simulink library "lib_fuel_converter3"  (Simulink 4.1.1)
values from neighbouring files (symbols this model uses):
  logFlag = 1    [advSACompMaskInit.m]    (also in advSACompMaskInitR13.m)
undefined symbols (not defined in the file or in its folder): air_cp, amb_tmp, cyc_mph, ex_gas_cp, fc_acc_mass, fc_base_mass, fc_c2i_th_cond, fc_c_init_tmp, fc_cl2h_eff, fc_CO2_to_FUELgps, fc_cold, fc_cold_tmp, fc_cp, fc_ct_trq, fc_emisv, fc_ext_sarea, fc_fuel_den, fc_fuel_lhv, fc_h2x_th_cond, fc_h_air_flow, fc_h_cp, fc_h_init_tmp, fc_hood_emisv, fc_hood_sarea, fc_i2x_th_cond, fc_i_init_tmp, fc_inertia, fc_map_spd, fc_map_trq, fc_max_trq, fc_nn_model_name, fc_pwr_scale, fc_spd_scale, fc_trq_scale, fc_tstat, fc_x_init_tmp, fd_ratio, gb_num_init, gb_ratio, generalName, pow, vc_idle_bool, vc_idle_spd, vc_key_on, veh_glider_mass, wh_radius
libraries: lib_fuel_converter3 x4, lib_etc x4, lib_fuel_converter x2, lib_fuel_converter2 x1
(part 4 of 9)

== system lib_fuel_converter3/configurable subsystems/fuel use and EO emis/fc temp/old fc coolant  temp. (C) ==
  fc on? : Inport  Port=1  LatchInput=off
  veh spd : Inport  Port=2  LatchInput=off
  Block NOTES : Subsystem
      settings: RTWFcnNameOpts=Auto  RTWFileNameOpts=Auto
      mask Display: disp('Block\nNOTES')
  Mux : Mux  Inputs=4
      settings: DisplayOption=none
  TEC : Integrator  ExternalReset=none  InitialConditionSource=internal  InitialCondition=fc_i_init_tmp  LimitOutput=off  UpperSaturationLimit=inf  LowerSaturationLimit=-inf  ShowSaturationPort=off  ShowStatePort=off  AbsoluteTolerance=auto
  compute engine dT/dt : Fcn  Expr=1.1*u[1]*(-u[2]/218)*(95-u[4])+(1-u[1])*u[3]*(u[4]-amb_tmp)
  gamma (takes v as input) : Fcn  Expr=(-8.22e-5*u+8.09e-6*4-1.45e-4)*.45
  log(1-40/75) : Constant  Value=-0.7621
  fc coolant  temp (C) : Outport  Port=1  InitialOutput=0
  wires:
  compute engine dT/dt/1 -> TEC/1
  gamma (takes v as input)/1 -> Mux/3
  log(1-40/75)/1 -> Mux/2
  Mux/1 -> compute engine dT/dt/1
  fc on?/1 -> Mux/1
  veh spd/1 -> gamma (takes v as input)/1
  TEC/1 -> fc coolant  temp (C)/1, Mux/4

== system lib_fuel_converter3/configurable subsystems/fuel use and EO emis/fc temp correct/fc temp correct Constant Correction Factors (Equation Based) ==
  Coolant T (C) : Inport  Port=1  LatchInput=off
  HOT fuel use (g/s) : Inport  Port=2  LatchInput=off
  HOT emis (g/s) : Inport  Port=3  LatchInput=off
  Enable : EnablePort  StatesWhenEnabling=reset
  Block NOTES : Subsystem
      settings: RTWFcnNameOpts=Auto  RTWFileNameOpts=Auto
      mask Display: disp('Block\nNOTES')
  CO cold/hot : Fcn  Expr=2.13*pow(u,4.26)+1
  HC cold/hot : Fcn  Expr=8.05*pow(u,9.46)+1
  Mux : Mux  Inputs=4
      settings: DisplayOption=none
  NOx cold/hot : Fcn  Expr=0.51*pow(u,1.37)+1
  PM cold/hot : Fcn  Expr=5.14*pow(u,17.04)+1
  Product : Product  Inputs=2  Multiplication=Element-wise(.*)  SaturateOnIntegerOverflow=on
  Product1 : Product  Inputs=2  Multiplication=Element-wise(.*)  SaturateOnIntegerOverflow=on
  Saturation : Saturate  UpperLimit=1  LowerLimit=0  LinearizeAsGain=on
  fuel cold/hot : Fcn  Expr=0.1*pow(u,0.65)+1
  lambda : Fcn  Expr=(fc_tstat-u)/(fc_tstat-20)
  fuel use (g/s) : Outport  Port=1  OutputWhenDisabled=reset  InitialOutput=0
  EO emis (g/s) : Outport  Port=2  OutputWhenDisabled=reset  InitialOutput=0
  wires:
  PM cold/hot/1 -> Mux/4
  NOx cold/hot/1 -> Mux/3
  HC cold/hot/1 -> Mux/1
  Saturation/1 -> CO cold/hot/1, HC cold/hot/1, fuel cold/hot/1, NOx cold/hot/1, PM cold/hot/1
  lambda/1 -> Saturation/1
  Mux/1 -> Product/1
  fuel cold/hot/1 -> Product1/2
  Product/1 -> EO emis (g/s)/1
  CO cold/hot/1 -> Mux/2
  Product1/1 -> fuel use (g/s)/1
  HOT fuel use (g/s)/1 -> Product1/1
  Coolant T (C)/1 -> lambda/1
  HOT emis (g/s)/1 -> Product/2

== system lib_fuel_converter3/configurable subsystems/fuel use and EO emis/fc temp correct/fc temp correct Variable Correction Factors (Map Based) ==
  Coolant T (C) : Inport  Port=1  LatchInput=off
  HOT fuel use (g/s) : Inport  Port=2  LatchInput=off
  HOT emis (g/s) : Inport  Port=3  LatchInput=off
  T (Nm) : Inport  Port=4  LatchInput=off
  w (rad/s) : Inport  Port=5  LatchInput=off
  Enable : EnablePort  StatesWhenEnabling=reset
  (Thot-Temp) -------------------- (Thot-Tcold) : Fcn  Expr=(fc_tstat-u)/(fc_tstat-fc_cold_tmp)
  CO factor cold-to-hot : Subsystem  mask(2-D Table Lookup){@1=fc_map_spd*fc_spd_scale, @2=fc_map_trq*fc_trq_scale, @3=fc_co_map_c2h}
      mask prompts: @1 "X Index"; @2 "Y Index"; @3 "Table"
      mask help:
      | Two Dimensional Table Lookup
      | The first input corresponds to X Index and the second input corresponds to the Y Index
      mask init:
      | xindex=@1; yindex=@2; table=@3; sftab2chk(xindex,yindex,table);
      settings: RTWFcnNameOpts=Auto  RTWFileNameOpts=Auto
      mask Help: This block returns a linearly interpolated intersection from the table using the X index (which corresponds to the rows of the table) and the Y index (which corresponds to the columns of the table).  Extrapolation is used.
      mask Display: plot(-10,-10,110,110,[90,50,10],[90,40,30],[90,50,10],[50,26,20],[90,50,10],[22,13,10])
  HC factor cold-to-hot : Subsystem  mask(2-D Table Lookup){@1=fc_map_spd*fc_spd_scale, @2=fc_map_trq*fc_trq_scale, @3=fc_hc_map_c2h}
      mask prompts: @1 "X Index"; @2 "Y Index"; @3 "Table"
      mask help:
      | Two Dimensional Table Lookup
      | The first input corresponds to X Index and the second input corresponds to the Y Index
      mask init:
      | xindex=@1; yindex=@2; table=@3; sftab2chk(xindex,yindex,table);
      settings: RTWFcnNameOpts=Auto  RTWFileNameOpts=Auto
      mask Help: This block returns a linearly interpolated intersection from the table using the X index (which corresponds to the rows of the table) and the Y index (which corresponds to the columns of the table).  Extrapolation is used.
      mask Display: plot(-10,-10,110,110,[90,50,10],[90,40,30],[90,50,10],[50,26,20],[90,50,10],[22,13,10])
  Mux{1..5} (5 alike) : Mux  Inputs=2
      settings: DisplayOption=none
  Mux6 : Mux  Inputs=4
      settings: DisplayOption=none
  NOx factor cold-to-hot : Subsystem  mask(2-D Table Lookup){@1=fc_map_spd*fc_spd_scale, @2=fc_map_trq*fc_trq_scale, @3=fc_nox_map_c2h}
      mask prompts: @1 "X Index"; @2 "Y Index"; @3 "Table"
      mask help:
      | Two Dimensional Table Lookup
      | The first input corresponds to X Index and the second input corresponds to the Y Index
      mask init:
      | xindex=@1; yindex=@2; table=@3; sftab2chk(xindex,yindex,table);
      settings: RTWFcnNameOpts=Auto  RTWFileNameOpts=Auto
      mask Help: This block returns a linearly interpolated intersection from the table using the X index (which corresponds to the rows of the table) and the Y index (which corresponds to the columns of the table).  Extrapolation is used.
      mask Display: plot(-10,-10,110,110,[90,50,10],[90,40,30],[90,50,10],[50,26,20],[90,50,10],[22,13,10])
  PM factor cold-to-hot : Subsystem  mask(2-D Table Lookup){@1=fc_map_spd*fc_spd_scale, @2=fc_map_trq*fc_trq_scale, @3=fc_pm_map_c2h}
      mask prompts: @1 "X Index"; @2 "Y Index"; @3 "Table"
      mask help:
      | Two Dimensional Table Lookup
      | The first input corresponds to X Index and the second input corresponds to the Y Index
      mask init:
      | xindex=@1; yindex=@2; table=@3; sftab2chk(xindex,yindex,table);
      settings: RTWFcnNameOpts=Auto  RTWFileNameOpts=Auto
      mask Help: This block returns a linearly interpolated intersection from the table using the X index (which corresponds to the rows of the table) and the Y index (which corresponds to the columns of the table).  Extrapolation is used.
      mask Display: plot(-10,-10,110,110,[90,50,10],[90,40,30],[90,50,10],[50,26,20],[90,50,10],[22,13,10])
  Product : Product  Inputs=2  Multiplication=Element-wise(.*)  SaturateOnIntegerOverflow=on
  Product1 : Product  Inputs=2  Multiplication=Element-wise(.*)  SaturateOnIntegerOverflow=on
  Saturation1 : Saturate  UpperLimit=max(fc_map_trq*fc_trq_scale)  LowerLimit=min(fc_map_trq*fc_trq_scale)  LinearizeAsGain=on
  Saturation2 : Saturate  UpperLimit=max(fc_map_spd*fc_spd_scale)  LowerLimit=min(fc_map_spd*fc_spd_scale)  LinearizeAsGain=on
  cold/hot =1+(factor-1) *Temp_ratio{,1..4} (5 alike) : Fcn  Expr=1+(u[2]-1)*u[1]
  fuel factor cold-to-hot : Subsystem  mask(2-D Table Lookup){@1=fc_map_spd*fc_spd_scale, @2=fc_map_trq*fc_trq_scale, @3=fc_fuel_map_c2h}
      mask prompts: @1 "X Index"; @2 "Y Index"; @3 "Table"
      mask help:
      | Two Dimensional Table Lookup
      | The first input corresponds to X Index and the second input corresponds to the Y Index
      mask init:
      | xindex=@1; yindex=@2; table=@3; sftab2chk(xindex,yindex,table);
      settings: RTWFcnNameOpts=Auto  RTWFileNameOpts=Auto
      mask Help: This block returns a linearly interpolated intersection from the table using the X index (which corresponds to the rows of the table) and the Y index (which corresponds to the columns of the table).  Extrapolation is used.
      mask Display: plot(-10,-10,110,110,[90,50,10],[90,40,30],[90,50,10],[50,26,20],[90,50,10],[22,13,10])
  limit to data limits : Saturate  UpperLimit=1  LowerLimit=0  LinearizeAsGain=on
  fuel use (g/s) : Outport  Port=1  OutputWhenDisabled=reset  InitialOutput=0
  EO emis (g/s) : Outport  Port=2  OutputWhenDisabled=reset  InitialOutput=0
  wires:
  cold/hot =1+(factor-1) *Temp_ratio4/1 -> Mux6/4
  cold/hot =1+(factor-1) *Temp_ratio3/1 -> Mux6/3
  cold/hot =1+(factor-1) *Temp_ratio2/1 -> Mux6/2
  cold/hot =1+(factor-1) *Temp_ratio1/1 -> Mux6/1
  cold/hot =1+(factor-1) *Temp_ratio/1 -> Product1/2
  limit to data limits/1 -> Mux5/1, Mux4/1, Mux3/1, Mux2/1, Mux1/1
  (Thot-Temp) -------------------- (Thot-Tcold)/1 -> limit to data limits/1
  Mux6/1 -> Product/1
  w (rad/s)/1 -> Saturation2/1
  T (Nm)/1 -> Saturation1/1
  HOT emis (g/s)/1 -> Product/2
  Product/1 -> EO emis (g/s)/1
  Product1/1 -> fuel use (g/s)/1
  Mux5/1 -> cold/hot =1+(factor-1) *Temp_ratio4/1
  Mux4/1 -> cold/hot =1+(factor-1) *Temp_ratio3/1
  Mux3/1 -> cold/hot =1+(factor-1) *Temp_ratio2/1
  Mux2/1 -> cold/hot =1+(factor-1) *Temp_ratio1/1
  PM factor cold-to-hot/1(table out) -> Mux5/2
  NOx factor cold-to-hot/1(table out) -> Mux4/2
  CO factor cold-to-hot/1(table out) -> Mux3/2
  HC factor cold-to-hot/1(table out) -> Mux2/2
  Mux1/1 -> cold/hot =1+(factor-1) *Temp_ratio/1
  fuel factor cold-to-hot/1(table out) -> Mux1/2
  Coolant T (C)/1 -> (Thot-Temp) -------------------- (Thot-Tcold)/1
  Saturation1/1 -> PM factor cold-to-hot/2(y0), NOx factor cold-to-hot/2(y0), CO factor cold-to-hot/2(y0), HC factor cold-to-hot/2(y0), fuel factor cold-to-hot/2(y0)
  Saturation2/1 -> PM factor cold-to-hot/1(x0), NOx factor cold-to-hot/1(x0), CO factor cold-to-hot/1(x0), HC factor cold-to-hot/1(x0), fuel factor cold-to-hot/1(x0)
  HOT fuel use (g/s)/1 -> Product1/1

== system lib_fuel_converter3/configurable subsystems/fuel use and EO emis Neural Network Model/HOT engine maps/Block NOTES ==
  note: This block determines the fully hot fuel use, engine-out emissions output rates, exhaust gas mass flow rate,
      | and engine-out exhaust gas temperature as a function of engine output torque and speed.
      | The engine maps (except for exhaust gas temperature) can be scaled using variables fc_spd_scale and
      |  fc_trq_scale; it is recommended that scaling values outside the range of 0.85 to 1.15 be used CAREFULLY.

== system lib_fuel_converter3/configurable subsystems/fuel use and EO emis Neural Network Model/HOT engine maps/CO (g/s) ==
  x0 : Inport  Port=1  LatchInput=off
  y0 : Inport  Port=2  LatchInput=off
  Mux : Mux  Inputs=2
      settings: DisplayOption=none
  S-function : S-Function  FunctionName=sftable2  Parameters=xindex, yindex, table  PortCounts=[]  SFunctionModules=''
  table out : Outport  Port=1  InitialOutput=0
  wires:
  y0/1 -> Mux/2
  S-function/1 -> table out/1
  x0/1 -> Mux/1
  Mux/1 -> S-function/1

== system lib_fuel_converter3/configurable subsystems/fuel use and EO emis Neural Network Model/HOT engine maps/HC (g/s) ==
  x0 : Inport  Port=1  LatchInput=off
  y0 : Inport  Port=2  LatchInput=off
  Mux : Mux  Inputs=2
      settings: DisplayOption=none
  S-function : S-Function  FunctionName=sftable2  Parameters=xindex, yindex, table  PortCounts=[]  SFunctionModules=''
  table out : Outport  Port=1  InitialOutput=0
  wires:
  y0/1 -> Mux/2
  S-function/1 -> table out/1
  x0/1 -> Mux/1
  Mux/1 -> S-function/1

== system lib_fuel_converter3/configurable subsystems/fuel use and EO emis Neural Network Model/HOT engine maps/MF,ex (g/s) ==
  x0 : Inport  Port=1  LatchInput=off
  y0 : Inport  Port=2  LatchInput=off
  Mux : Mux  Inputs=2
      settings: DisplayOption=none
  S-function : S-Function  FunctionName=sftable2  Parameters=xindex, yindex, table  PortCounts=[]  SFunctionModules=''
  table out : Outport  Port=1  InitialOutput=0
  wires:
  y0/1 -> Mux/2
  S-function/1 -> table out/1
  x0/1 -> Mux/1
  Mux/1 -> S-function/1

== system lib_fuel_converter3/configurable subsystems/fuel use and EO emis Neural Network Model/HOT engine maps/NOx (g/s) ==
  x0 : Inport  Port=1  LatchInput=off
  y0 : Inport  Port=2  LatchInput=off
  Mux : Mux  Inputs=2
      settings: DisplayOption=none
  S-function : S-Function  FunctionName=sftable2  Parameters=xindex, yindex, table  PortCounts=[]  SFunctionModules=''
  table out : Outport  Port=1  InitialOutput=0
  wires:
  y0/1 -> Mux/2
  S-function/1 -> table out/1
  x0/1 -> Mux/1
  Mux/1 -> S-function/1

== system lib_fuel_converter3/configurable subsystems/fuel use and EO emis Neural Network Model/HOT engine maps/O2 (g/s) ==
  x0 : Inport  Port=1  LatchInput=off
  y0 : Inport  Port=2  LatchInput=off
  Mux : Mux  Inputs=2
      settings: DisplayOption=none
  S-function : S-Function  FunctionName=sftable2  Parameters=xindex, yindex, table  PortCounts=[]  SFunctionModules=''
  table out : Outport  Port=1  InitialOutput=0
  wires:
  Mux/1 -> S-function/1
  x0/1 -> Mux/1
  S-function/1 -> table out/1
  y0/1 -> Mux/2

== system lib_fuel_converter3/configurable subsystems/fuel use and EO emis Neural Network Model/HOT engine maps/PM (g/s) ==
  x0 : Inport  Port=1  LatchInput=off
  y0 : Inport  Port=2  LatchInput=off
  Mux : Mux  Inputs=2
      settings: DisplayOption=none
  S-function : S-Function  FunctionName=sftable2  Parameters=xindex, yindex, table  PortCounts=[]  SFunctionModules=''
  table out : Outport  Port=1  InitialOutput=0
  wires:
  y0/1 -> Mux/2
  S-function/1 -> table out/1
  x0/1 -> Mux/1
  Mux/1 -> S-function/1

== system lib_fuel_converter3/configurable subsystems/fuel use and EO emis Neural Network Model/HOT engine maps/Tex,eo (C) ==
  x0 : Inport  Port=1  LatchInput=off
  y0 : Inport  Port=2  LatchInput=off
  Mux : Mux  Inputs=2
      settings: DisplayOption=none
  S-function : S-Function  FunctionName=sftable2  Parameters=xindex, yindex, table  PortCounts=[]  SFunctionModules=''
  table out : Outport  Port=1  InitialOutput=0
  wires:
  y0/1 -> Mux/2
  S-function/1 -> table out/1
  x0/1 -> Mux/1
  Mux/1 -> S-function/1

== system lib_fuel_converter3/configurable subsystems/fuel use and EO emis Neural Network Model/HOT engine maps/fuel (g/s) ==
  x0 : Inport  Port=1  LatchInput=off
  y0 : Inport  Port=2  LatchInput=off
  Mux : Mux  Inputs=2
      settings: DisplayOption=none
  S-function : S-Function  FunctionName=sftable2  Parameters=xindex, yindex, table  PortCounts=[]  SFunctionModules=''
  table out : Outport  Port=1  InitialOutput=0
  wires:
  y0/1 -> Mux/2
  S-function/1 -> table out/1
  x0/1 -> Mux/1
  Mux/1 -> S-function/1

== system lib_fuel_converter3/configurable subsystems/fuel use and EO emis Neural Network Model/fc temp/Block NOTES ==
  note: This block models the thermal behavior internal combustion engine (ICE).
      | Emphasis is on the coolant since this temperature is used to correct engine
      | fuel use.

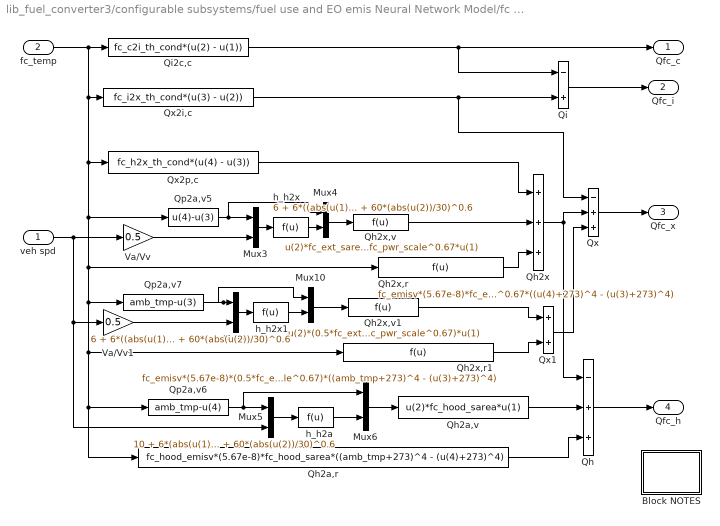
== system lib_fuel_converter3/configurable subsystems/fuel use and EO emis Neural Network Model/fc temp/fc mass heat flow ==
  veh spd : Inport  Port=1  LatchInput=off
  fc_temp : Inport  Port=2  LatchInput=off
  Block NOTES : Subsystem
      settings: RTWFcnNameOpts=Auto  RTWFileNameOpts=Auto
      mask Display: disp('Block\nNOTES')
  Mux{3..6,9..10} (6 alike) : Mux  Inputs=2
      settings: DisplayOption=none
  Qh : Sum  Inputs=-++  SaturateOnIntegerOverflow=on
  Qh2a,r : Fcn  Expr=fc_hood_emisv*(5.67e-8)*fc_hood_sarea*((amb_tmp+273)^4 - (u(4)+273)^4)
  Qh2a,v : Fcn  Expr=u(2)*fc_hood_sarea*u(1)
  Qh2x : Sum  Inputs=+++  SaturateOnIntegerOverflow=on
  Qh2x,r : Fcn  Expr=fc_emisv*(5.67e-8)*fc_ext_sarea*fc_pwr_scale^0.67*((u(4)+273)^4 - (u(3)+273)^4)
  Qh2x,r1 : Fcn  Expr=fc_emisv*(5.67e-8)*(0.5*fc_ext_sarea*fc_pwr_scale^0.67)*((amb_tmp+273)^4 - (u(3)+273)^4)
  Qh2x,v : Fcn  Expr=u(2)*fc_ext_sarea*fc_pwr_scale^0.67*u(1)
  Qh2x,v1 : Fcn  Expr=u(2)*(0.5*fc_ext_sarea*fc_pwr_scale^0.67)*u(1)
  Qi : Sum  Inputs=-+  SaturateOnIntegerOverflow=on
  Qi2c,c : Fcn  Expr=fc_c2i_th_cond*(u(2) - u(1))
  Qp2a,v5 : Fcn  Expr=u(4)-u(3)
  Qp2a,v6 : Fcn  Expr=amb_tmp-u(4)
  Qp2a,v7 : Fcn  Expr=amb_tmp-u(3)
  Qx : Sum  Inputs=-++  SaturateOnIntegerOverflow=on
  Qx1 : Sum  Inputs=++  SaturateOnIntegerOverflow=on
  Qx2i,c : Fcn  Expr=fc_i2x_th_cond*(u(3) - u(2))
  Qx2p,c : Fcn  Expr=fc_h2x_th_cond*(u(4) - u(3))
  Va/Vv : Gain  Gain=0.5  Multiplication=Element-wise(K.*u)  SaturateOnIntegerOverflow=on
  Va/Vv1 : Gain  Gain=0.5  Multiplication=Element-wise(K.*u)  SaturateOnIntegerOverflow=on
  h_h2a : Fcn  Expr=10 + 6*(abs(u(1))/1000)^0.3 + 60*(abs(u(2))/30)^0.6
  h_h2x : Fcn  Expr=6 + 6*((abs(u(1))/1000))^0.3 + 60*(abs(u(2))/30)^0.6
  h_h2x1 : Fcn  Expr=6 + 6*((abs(u(1))/1000))^0.3 + 60*(abs(u(2))/30)^0.6
  Qfc_c : Outport  Port=1
  Qfc_i : Outport  Port=2
  Qfc_x : Outport  Port=3
  Qfc_h : Outport  Port=4
  wires:
  Mux10/1 -> Qh2x,v1/1
  Mux9/1 -> h_h2x1/1
  Qp2a,v7/1 -> Mux9/1, Mux10/1
  h_h2x1/1 -> Mux10/2
  Va/Vv1/1 -> Mux9/2
  Mux4/1 -> Qh2x,v/1
  Mux3/1 -> h_h2x/1
  Qp2a,v5/1 -> Mux3/1, Mux4/1
  h_h2x/1 -> Mux4/2
  veh spd/1 -> Va/Vv/1, Mux5/2, Va/Vv1/1
  Va/Vv/1 -> Mux3/2
  Qi2c,c/1 -> Qfc_c/1, Qi/1
  fc_temp/1 -> Qx2p,c/1, Qh2x,r/1, Qp2a,v7/1, Qp2a,v6/1, Qh2a,r/1, Qh2x,r1/1, Qp2a,v5/1, Qx2i,c/1, Qi2c,c/1
  Qx2i,c/1 -> Qi/2, Qx/1
  Qi/1 -> Qfc_i/1
  Qx/1 -> Qfc_x/1
  Qh2x/1 -> Qx/2, Qh/1
  Qh/1 -> Qfc_h/1
  Mux6/1 -> Qh2a,v/1
  Mux5/1 -> h_h2a/1
  Qp2a,v6/1 -> Mux5/1, Mux6/1
  h_h2a/1 -> Mux6/2
  Qx1/1 -> Qx/3
  Qh2x,v/1 -> Qh2x/2
  Qx2p,c/1 -> Qh2x/1
  Qh2x,r1/1 -> Qx1/2
  Qh2x,v1/1 -> Qx1/1
  Qh2a,r/1 -> Qh/3
  Qh2a,v/1 -> Qh/2
  Qh2x,r/1 -> Qh2x/3

== system lib_fuel_converter3/configurable subsystems/fuel use and EO emis Neural Network Model/fc temp/old fc coolant  temp. (C) ==
  fc on? : Inport  Port=1  LatchInput=off
  veh spd : Inport  Port=2  LatchInput=off
  Block NOTES : Subsystem
      settings: RTWFcnNameOpts=Auto  RTWFileNameOpts=Auto
      mask Display: disp('Block\nNOTES')
  Mux : Mux  Inputs=4
      settings: DisplayOption=none
  TEC : Integrator  ExternalReset=none  InitialConditionSource=internal  InitialCondition=fc_i_init_tmp  LimitOutput=off  UpperSaturationLimit=inf  LowerSaturationLimit=-inf  ShowSaturationPort=off  ShowStatePort=off  AbsoluteTolerance=auto
  compute engine dT/dt : Fcn  Expr=1.1*u[1]*(-u[2]/218)*(95-u[4])+(1-u[1])*u[3]*(u[4]-amb_tmp)
  gamma (takes v as input) : Fcn  Expr=(-8.22e-5*u+8.09e-6*4-1.45e-4)*.45
  log(1-40/75) : Constant  Value=-0.7621
  fc coolant  temp (C) : Outport  Port=1  InitialOutput=0
  wires:
  compute engine dT/dt/1 -> TEC/1
  gamma (takes v as input)/1 -> Mux/3
  log(1-40/75)/1 -> Mux/2
  Mux/1 -> compute engine dT/dt/1
  fc on?/1 -> Mux/1
  veh spd/1 -> gamma (takes v as input)/1
  TEC/1 -> fc coolant  temp (C)/1, Mux/4

== system lib_fuel_converter3/configurable subsystems/fuel use and EO emis Neural Network Model/fc temp correct/fc temp correct Constant Correction Factors (Equation Based) ==
  Coolant T (C) : Inport  Port=1  LatchInput=off
  HOT fuel use (g/s) : Inport  Port=2  LatchInput=off
  HOT emis (g/s) : Inport  Port=3  LatchInput=off
  Enable : EnablePort  StatesWhenEnabling=reset
  Block NOTES : Subsystem
      settings: RTWFcnNameOpts=Auto  RTWFileNameOpts=Auto
      mask Display: disp('Block\nNOTES')
  CO cold/hot : Fcn  Expr=2.13*pow(u,4.26)+1
  HC cold/hot : Fcn  Expr=8.05*pow(u,9.46)+1
  Mux : Mux  Inputs=4
      settings: DisplayOption=none
  NOx cold/hot : Fcn  Expr=0.51*pow(u,1.37)+1
  PM cold/hot : Fcn  Expr=5.14*pow(u,17.04)+1
  Product : Product  Inputs=2  Multiplication=Element-wise(.*)  SaturateOnIntegerOverflow=on
  Product1 : Product  Inputs=2  Multiplication=Element-wise(.*)  SaturateOnIntegerOverflow=on
  Saturation : Saturate  UpperLimit=1  LowerLimit=0  LinearizeAsGain=on
  fuel cold/hot : Fcn  Expr=0.1*pow(u,0.65)+1
  lambda : Fcn  Expr=(fc_tstat-u)/(fc_tstat-20)
  fuel use (g/s) : Outport  Port=1  OutputWhenDisabled=reset  InitialOutput=0
  EO emis (g/s) : Outport  Port=2  OutputWhenDisabled=reset  InitialOutput=0
  wires:
  PM cold/hot/1 -> Mux/4
  NOx cold/hot/1 -> Mux/3
  HC cold/hot/1 -> Mux/1
  Saturation/1 -> CO cold/hot/1, HC cold/hot/1, fuel cold/hot/1, NOx cold/hot/1, PM cold/hot/1
  lambda/1 -> Saturation/1
  Mux/1 -> Product/1
  fuel cold/hot/1 -> Product1/2
  Product/1 -> EO emis (g/s)/1
  CO cold/hot/1 -> Mux/2
  Product1/1 -> fuel use (g/s)/1
  HOT fuel use (g/s)/1 -> Product1/1
  Coolant T (C)/1 -> lambda/1
  HOT emis (g/s)/1 -> Product/2

== system lib_fuel_converter3/configurable subsystems/fuel use and EO emis Neural Network Model/fc temp correct/fc temp correct Variable Correction Factors (Map Based) ==
  Coolant T (C) : Inport  Port=1  LatchInput=off
  HOT fuel use (g/s) : Inport  Port=2  LatchInput=off
  HOT emis (g/s) : Inport  Port=3  LatchInput=off
  T (Nm) : Inport  Port=4  LatchInput=off
  w (rad/s) : Inport  Port=5  LatchInput=off
  Enable : EnablePort  StatesWhenEnabling=reset
  (Thot-Temp) -------------------- (Thot-Tcold) : Fcn  Expr=(fc_tstat-u)/(fc_tstat-fc_cold_tmp)
  CO factor cold-to-hot : Subsystem  mask(2-D Table Lookup){@1=fc_map_spd*fc_spd_scale, @2=fc_map_trq*fc_trq_scale, @3=fc_co_map_c2h}
      mask prompts: @1 "X Index"; @2 "Y Index"; @3 "Table"
      mask help:
      | Two Dimensional Table Lookup
      | The first input corresponds to X Index and the second input corresponds to the Y Index
      mask init:
      | xindex=@1; yindex=@2; table=@3; sftab2chk(xindex,yindex,table);
      settings: RTWFcnNameOpts=Auto  RTWFileNameOpts=Auto
      mask Help: This block returns a linearly interpolated intersection from the table using the X index (which corresponds to the rows of the table) and the Y index (which corresponds to the columns of the table).  Extrapolation is used.
      mask Display: plot(-10,-10,110,110,[90,50,10],[90,40,30],[90,50,10],[50,26,20],[90,50,10],[22,13,10])
  HC factor cold-to-hot : Subsystem  mask(2-D Table Lookup){@1=fc_map_spd*fc_spd_scale, @2=fc_map_trq*fc_trq_scale, @3=fc_hc_map_c2h}
      mask prompts: @1 "X Index"; @2 "Y Index"; @3 "Table"
      mask help:
      | Two Dimensional Table Lookup
      | The first input corresponds to X Index and the second input corresponds to the Y Index
      mask init:
      | xindex=@1; yindex=@2; table=@3; sftab2chk(xindex,yindex,table);
      settings: RTWFcnNameOpts=Auto  RTWFileNameOpts=Auto
      mask Help: This block returns a linearly interpolated intersection from the table using the X index (which corresponds to the rows of the table) and the Y index (which corresponds to the columns of the table).  Extrapolation is used.
      mask Display: plot(-10,-10,110,110,[90,50,10],[90,40,30],[90,50,10],[50,26,20],[90,50,10],[22,13,10])
  Mux{1..5} (5 alike) : Mux  Inputs=2
      settings: DisplayOption=none
  Mux6 : Mux  Inputs=4
      settings: DisplayOption=none
  NOx factor cold-to-hot : Subsystem  mask(2-D Table Lookup){@1=fc_map_spd*fc_spd_scale, @2=fc_map_trq*fc_trq_scale, @3=fc_nox_map_c2h}
      mask prompts: @1 "X Index"; @2 "Y Index"; @3 "Table"
      mask help:
      | Two Dimensional Table Lookup
      | The first input corresponds to X Index and the second input corresponds to the Y Index
      mask init:
      | xindex=@1; yindex=@2; table=@3; sftab2chk(xindex,yindex,table);
      settings: RTWFcnNameOpts=Auto  RTWFileNameOpts=Auto
      mask Help: This block returns a linearly interpolated intersection from the table using the X index (which corresponds to the rows of the table) and the Y index (which corresponds to the columns of the table).  Extrapolation is used.
      mask Display: plot(-10,-10,110,110,[90,50,10],[90,40,30],[90,50,10],[50,26,20],[90,50,10],[22,13,10])
  PM factor cold-to-hot : Subsystem  mask(2-D Table Lookup){@1=fc_map_spd*fc_spd_scale, @2=fc_map_trq*fc_trq_scale, @3=fc_pm_map_c2h}
      mask prompts: @1 "X Index"; @2 "Y Index"; @3 "Table"
      mask help:
      | Two Dimensional Table Lookup
      | The first input corresponds to X Index and the second input corresponds to the Y Index
      mask init:
      | xindex=@1; yindex=@2; table=@3; sftab2chk(xindex,yindex,table);
      settings: RTWFcnNameOpts=Auto  RTWFileNameOpts=Auto
      mask Help: This block returns a linearly interpolated intersection from the table using the X index (which corresponds to the rows of the table) and the Y index (which corresponds to the columns of the table).  Extrapolation is used.
      mask Display: plot(-10,-10,110,110,[90,50,10],[90,40,30],[90,50,10],[50,26,20],[90,50,10],[22,13,10])
  Product : Product  Inputs=2  Multiplication=Element-wise(.*)  SaturateOnIntegerOverflow=on
  Product1 : Product  Inputs=2  Multiplication=Element-wise(.*)  SaturateOnIntegerOverflow=on
  Saturation1 : Saturate  UpperLimit=max(fc_map_trq*fc_trq_scale)  LowerLimit=min(fc_map_trq*fc_trq_scale)  LinearizeAsGain=on
  Saturation2 : Saturate  UpperLimit=max(fc_map_spd*fc_spd_scale)  LowerLimit=min(fc_map_spd*fc_spd_scale)  LinearizeAsGain=on
  cold/hot =1+(factor-1) *Temp_ratio{,1..4} (5 alike) : Fcn  Expr=1+(u[2]-1)*u[1]
  fuel factor cold-to-hot : Subsystem  mask(2-D Table Lookup){@1=fc_map_spd*fc_spd_scale, @2=fc_map_trq*fc_trq_scale, @3=fc_fuel_map_c2h}
      mask prompts: @1 "X Index"; @2 "Y Index"; @3 "Table"
      mask help:
      | Two Dimensional Table Lookup
      | The first input corresponds to X Index and the second input corresponds to the Y Index
      mask init:
      | xindex=@1; yindex=@2; table=@3; sftab2chk(xindex,yindex,table);
      settings: RTWFcnNameOpts=Auto  RTWFileNameOpts=Auto
      mask Help: This block returns a linearly interpolated intersection from the table using the X index (which corresponds to the rows of the table) and the Y index (which corresponds to the columns of the table).  Extrapolation is used.
      mask Display: plot(-10,-10,110,110,[90,50,10],[90,40,30],[90,50,10],[50,26,20],[90,50,10],[22,13,10])
  limit to data limits : Saturate  UpperLimit=1  LowerLimit=0  LinearizeAsGain=on
  fuel use (g/s) : Outport  Port=1  OutputWhenDisabled=reset  InitialOutput=0
  EO emis (g/s) : Outport  Port=2  OutputWhenDisabled=reset  InitialOutput=0
  wires:
  cold/hot =1+(factor-1) *Temp_ratio4/1 -> Mux6/4
  cold/hot =1+(factor-1) *Temp_ratio3/1 -> Mux6/3
  cold/hot =1+(factor-1) *Temp_ratio2/1 -> Mux6/2
  cold/hot =1+(factor-1) *Temp_ratio1/1 -> Mux6/1
  cold/hot =1+(factor-1) *Temp_ratio/1 -> Product1/2
  limit to data limits/1 -> Mux5/1, Mux4/1, Mux3/1, Mux2/1, Mux1/1
  (Thot-Temp) -------------------- (Thot-Tcold)/1 -> limit to data limits/1
  Mux6/1 -> Product/1
  w (rad/s)/1 -> Saturation2/1
  T (Nm)/1 -> Saturation1/1
  HOT emis (g/s)/1 -> Product/2
  Product/1 -> EO emis (g/s)/1
  Product1/1 -> fuel use (g/s)/1
  Mux5/1 -> cold/hot =1+(factor-1) *Temp_ratio4/1
  Mux4/1 -> cold/hot =1+(factor-1) *Temp_ratio3/1
  Mux3/1 -> cold/hot =1+(factor-1) *Temp_ratio2/1
  Mux2/1 -> cold/hot =1+(factor-1) *Temp_ratio1/1
  PM factor cold-to-hot/1(table out) -> Mux5/2
  NOx factor cold-to-hot/1(table out) -> Mux4/2
  CO factor cold-to-hot/1(table out) -> Mux3/2
  HC factor cold-to-hot/1(table out) -> Mux2/2
  Mux1/1 -> cold/hot =1+(factor-1) *Temp_ratio/1
  fuel factor cold-to-hot/1(table out) -> Mux1/2
  Coolant T (C)/1 -> (Thot-Temp) -------------------- (Thot-Tcold)/1
  Saturation1/1 -> PM factor cold-to-hot/2(y0), NOx factor cold-to-hot/2(y0), CO factor cold-to-hot/2(y0), HC factor cold-to-hot/2(y0), fuel factor cold-to-hot/2(y0)
  Saturation2/1 -> PM factor cold-to-hot/1(x0), NOx factor cold-to-hot/1(x0), CO factor cold-to-hot/1(x0), HC factor cold-to-hot/1(x0), fuel factor cold-to-hot/1(x0)
  HOT fuel use (g/s)/1 -> Product1/1

== system lib_fuel_converter3/fuel converter  <fc> for series/Model & Interface/model/Block NOTES ==
  note: This block models the internal combustion engine, and includes inertia effects,
      | performance limits, accessory loads, and temperature transient effects on fuel
      | use, engine-out emissions, and catalyst efficiency.  There are 'leads' to the
      | engine controller here, which controller determines whether the engine is on.

== system lib_fuel_converter3/fuel converter  <fc> for series/Model & Interface/model/enhancedToWorkspace ==
  In1 : Inport  Port=1  LatchInput=off
  To Workspace : ToWorkspace  VariableName=fc_spd_out_r  SampleTime=-1  SaveFormat=Array
  wires:
  In1/1 -> To Workspace/1

== system lib_fuel_converter3/fuel converter  <fc> for series/Model & Interface/model/enhancedToWorkspace1 ==
  In1 : Inport  Port=1  LatchInput=off
  To Workspace : ToWorkspace  VariableName=fc_trq_out_r  SampleTime=-1  SaveFormat=Array
  wires:
  In1/1 -> To Workspace/1

== system lib_fuel_converter3/fuel converter  <fc> for series/Model & Interface/model/enhancedToWorkspace2 ==
  In1 : Inport  Port=1  LatchInput=off
  To Workspace : ToWorkspace  VariableName=fc_spd_est  SampleTime=-1  SaveFormat=Array
  wires:
  In1/1 -> To Workspace/1

== system lib_fuel_converter3/fuel converter  <fc> for series/Model & Interface/model/enhancedToWorkspace3 ==
  In1 : Inport  Port=1  LatchInput=off
  To Workspace : ToWorkspace  VariableName=fc_brake_trq  SampleTime=-1  SaveFormat=Array
  wires:
  In1/1 -> To Workspace/1

== system lib_fuel_converter3/fuel converter  <fc> for series/Model & Interface/model/fuel use and EO emis Configurable Subsystem ==
  T (Nm) : Inport  Port=1  LatchInput=off
  w (rad/s) : Inport  Port=2  LatchInput=off
  fuel use and EO emis : lib_fuel_converter3/configurable subsystems/fuel use and EO emis
      settings: RTWFcnNameOpts=Auto  RTWFileNameOpts=Auto
  cumulative fuel  use (gal) : Outport  Port=1
  "FC ON?, EOem, MFex, Tex, O2ex" : Outport  Port=2
  Vv,Tfc : Outport  Port=3
  wires:
  T (Nm)/1 -> fuel use and EO emis/1
  w (rad/s)/1 -> fuel use and EO emis/2
  fuel use and EO emis/1 -> cumulative fuel  use (gal)/1
  fuel use and EO emis/2 -> "FC ON?, EOem, MFex, Tex, O2ex"/1
  fuel use and EO emis/3 -> Vv,Tfc/1

== system lib_fuel_converter3/fuel converter  <fc> for series/Model & Interface/model/help ==

== system lib_fuel_converter3/fuel converter  <fc> for series/Model & Interface/model/providing trq (+ive or -ive) ==
  req'd trq (Nm) : Inport  Port=1  LatchInput=off
  req'd spd (rad/s) : Inport  Port=2  LatchInput=off
  prev engine spd (rad/s) : Inport  Port=3  LatchInput=off
  Mux3 : Mux  Inputs=3
      settings: DisplayOption=none
  Sum1 : Sum  Inputs=+-  SaturateOnIntegerOverflow=on
  Sum2 : Sum  Inputs=++  SaturateOnIntegerOverflow=on
  effect of inertia (Nm) : Subsystem
      settings: RTWFcnNameOpts=Auto  RTWFileNameOpts=Auto
  enforce engine limits : Subsystem
      settings: RTWFcnNameOpts=Auto  RTWFileNameOpts=Auto
  map trq (Nm) spd (rad/s) trq to drivetrain (Nm) : Outport  Port=1  InitialOutput=0
  wires:
  req'd spd (rad/s)/1 -> enforce engine limits/2(req'd engine spd (rad/s))
  Sum1/1 -> Mux3/3
  Mux3/1 -> map trq (Nm) spd (rad/s) trq to drivetrain (Nm)/1
  prev engine spd (rad/s)/1 -> effect of inertia (Nm)/2(prev spd)
  enforce engine limits/1(limited engine brake trq (Nm)) -> Mux3/1, Sum1/1
  enforce engine limits/2(limited engine spd (rad/s)) -> effect of inertia (Nm)/1(req'd spd (rad/s)), Mux3/2
  req'd trq (Nm)/1 -> Sum2/1
  effect of inertia (Nm)/1((Nm)) -> Sum1/2, Sum2/2
  Sum2/1 -> enforce engine limits/1(req'd engine trq (Nm))

== system lib_fuel_converter3/fuel converter  <fc> for series/Model & Interface/model/spinning up or spinning down ==
  spd command (rad/s) : Inport  Port=1  LatchInput=off
  engine disconnected from drivetrain : Inport  Port=2  LatchInput=off
  previous engine spd (rad/s) : Inport  Port=3  LatchInput=off
  Constant : Constant  Value=0
  Constant1 : Constant  Value=vc_idle_spd
  MinMax : MinMax  Function=min  Inputs=2
  MinMax1 : MinMax  Function=max  Inputs=2
  Mux3 : Mux  Inputs=3
      settings: DisplayOption=none
  Product : Product  Inputs=2  Multiplication=Element-wise(.*)  SaturateOnIntegerOverflow=on
  Product2 : Product  Inputs=2  Multiplication=Element-wise(.*)  SaturateOnIntegerOverflow=on
  Relational Operator : RelationalOperator  Operator=<=
  Sum : Sum  Inputs=|++  SaturateOnIntegerOverflow=on
  Sum1 : Sum  Inputs=|+-  SaturateOnIntegerOverflow=on
  Sum2 : Sum  Inputs=++  SaturateOnIntegerOverflow=on
  Switch: map torque : Switch  Threshold=eps
  T_closed throttle : Subsystem
      settings: RTWFcnNameOpts=Auto  RTWFileNameOpts=Auto
  T_max : Subsystem
      settings: RTWFcnNameOpts=Auto  RTWFileNameOpts=Auto
  alpha : Gain  Gain=1/(fc_inertia+eps)  Multiplication=Element-wise(K.*u)  SaturateOnIntegerOverflow=on
  dt : Subsystem
      settings: RTWFcnNameOpts=Auto  RTWFileNameOpts=Auto
  effect of inertia (Nm) : Subsystem
      settings: RTWFcnNameOpts=Auto  RTWFileNameOpts=Auto
  just started spin-down/spin-up : Subsystem
      settings: RTWFcnNameOpts=Auto  RTWFileNameOpts=Auto
  no-lag Reset Integrator : Subsystem  mask(No-lag Reset Integrator){@1=vc_idle_spd}
      mask prompts: @1 "Initial Value"
      mask help: No-lag Reset Integrator
      mask init:
      | initval=@1;
      settings: RTWFcnNameOpts=Auto  RTWFileNameOpts=Auto
      mask Help: Integrates first input using Euler technique.\nAt the time step that input 2 <> zero,\noutput is reset to input 3.
      mask Display: disp('1/s\nw/ reset\nno lag')
  map trq (Nm) spd (rad/s) trq to drivetrain (Nm) : Outport  Port=1  InitialOutput=0
  wires:
  [acc_mech_trq_est] -> Sum1/2
  Sum1/1 -> alpha/1
  [acc_mech_trq_est] -> Sum/2
  Sum/1 -> MinMax/2
  effect of inertia (Nm)/1((Nm)) -> Sum/1
  MinMax1/1 -> Mux3/2
  Product2/1 -> MinMax1/2
  [engine_on] -> Product2/2
  Constant1/1 -> Product2/1
  Constant/1 -> Mux3/3
  Mux3/1 -> map trq (Nm) spd (rad/s) trq to drivetrain (Nm)/1
  dt/1(out_1) -> Product/2
  Product/1 -> Sum2/1
  engine disconnected from drivetrain/1 -> just started spin-down/spin-up/1(state)
  Sum2/1 -> no-lag Reset Integrator/3(in_3)
  just started spin-down/spin-up/1(trigger) -> no-lag Reset Integrator/2(in_2)
  no-lag Reset Integrator/1(out_1) -> MinMax1/1
  spd command (rad/s)/1 -> effect of inertia (Nm)/1(req'd spd (rad/s)), Relational Operator/2
  previous engine spd (rad/s)/1 -> Sum2/2, Relational Operator/1, effect of inertia (Nm)/2(prev spd), T_max/1(w_APU), T_closed throttle/1(w_APU)
  alpha/1 -> no-lag Reset Integrator/1(in_1), Product/1
  Relational Operator/1 -> Switch: map torque/2
  Switch: map torque/1 -> Sum1/1, Mux3/1
  T_closed throttle/1(T_closed throttle) -> Switch: map torque/3
  MinMax/1 -> Switch: map torque/1
  T_max/1(T_max) -> MinMax/1

== system lib_fuel_converter3/fuel converter <fc>/IC Engine Model  &  Interface/ic engine model/Block NOTES ==
  note: This block models the internal combustion engine, and includes inertia effects,
      | performance limits, accessory loads, and temperature transient effects on fuel
      | use, engine-out emissions, and catalyst efficiency.  There are 'leads' to the
      | engine controller here, which controller determines whether the engine is on.

== system lib_fuel_converter3/fuel converter <fc>/IC Engine Model  &  Interface/ic engine model/Speed Limits ==
  Speed Requested : Inport  Port=1  LatchInput=off
  Constant : Constant  Value=0
  Speed Limits : Saturate  UpperLimit=max(fc_map_spd)*fc_spd_scale  LowerLimit=vc_idle_spd*vc_idle_bool  LinearizeAsGain=on
  "if engine is not on, speed is zero" : Switch  Threshold=0.5
  Limited Speed Request : Outport  Port=1
  wires:
  Speed Requested/1 -> Speed Limits/1
  Speed Limits/1 -> "if engine is not on, speed is zero"/1
  "if engine is not on, speed is zero"/1 -> Limited Speed Request/1
  [engine_on] -> "if engine is not on, speed is zero"/2
  Constant/1 -> "if engine is not on, speed is zero"/3

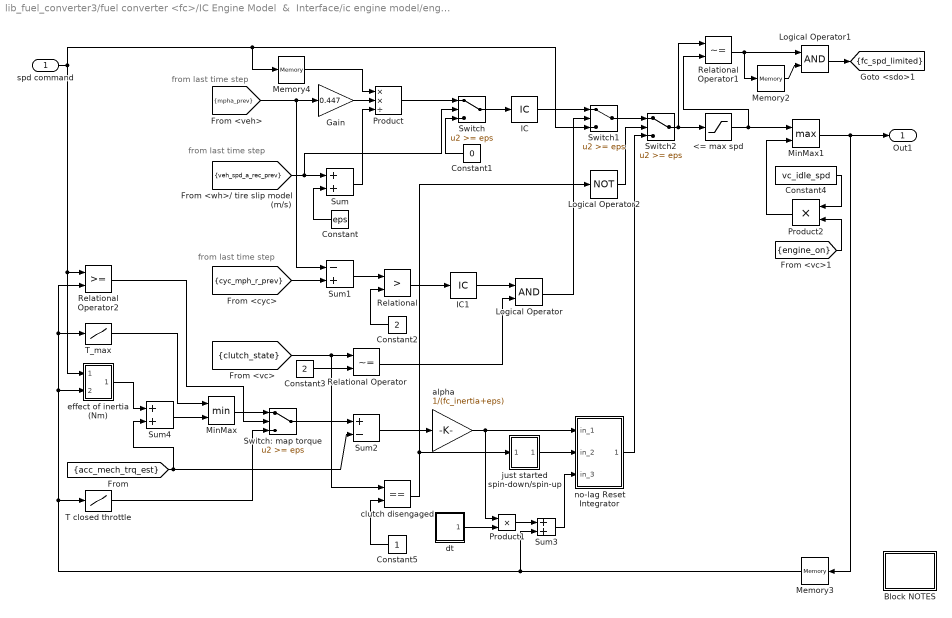
== system lib_fuel_converter3/fuel converter <fc>/IC Engine Model  &  Interface/ic engine model/engine speed estimator ==
  note: from last time step
  note: from last time step
  note: from last time step
  spd command : Inport  Port=1  LatchInput=off
  <= max spd : Saturate  UpperLimit=max(fc_map_spd)*fc_spd_scale  LowerLimit=-inf  LinearizeAsGain=on
  Block NOTES : Subsystem
      settings: RTWFcnNameOpts=Auto  RTWFileNameOpts=Auto
      mask Display: disp('Block\nNOTES')
  Constant : Constant  Orientation=left  Value=eps
  Constant1 : Constant  Orientation=left  Value=0
  Constant2 : Constant  Orientation=left  Value=2
  Constant3 : Constant  Value=2
  Constant4 : Constant  Value=vc_idle_spd
  Constant5 : Constant  Orientation=left  Value=1
  Gain : Gain  Gain=0.447  Multiplication=Element-wise(K.*u)  SaturateOnIntegerOverflow=on
  IC : InitialCondition  Value=cyc_mph(1,2)*0.447/wh_radius*fd_ratio*gb_ratio(gb_num_init)
  IC1 : InitialCondition  Value=0
  Logical Operator : Logic  Operator=AND  Inputs=2
  Logical Operator1 : Logic  Operator=AND  Inputs=2
  Logical Operator2 : Logic  Operator=NOT  Inputs=1
  Memory2 : Memory  X0=0  InheritSampleTime=off
      settings: RTWStateStorageClass=Auto
  Memory3 : Memory  Orientation=left  X0=cyc_mph(1,2)*0.447/wh_radius*fd_ratio*max(gb_ratio)  InheritSampleTime=off
      settings: RTWStateStorageClass=Auto
  Memory4 : Memory  X0=0  InheritSampleTime=off
      settings: RTWStateStorageClass=Auto
  MinMax : MinMax  Function=min  Inputs=2
  MinMax1 : MinMax  Function=max  Inputs=2
  Product : Product  Inputs=**/  Multiplication=Element-wise(.*)  SaturateOnIntegerOverflow=on
  Product1 : Product  Inputs=2  Multiplication=Element-wise(.*)  SaturateOnIntegerOverflow=on
  Product2 : Product  Orientation=left  Inputs=2  Multiplication=Element-wise(.*)  SaturateOnIntegerOverflow=on
  Relational : RelationalOperator  Operator=>
  Relational Operator : RelationalOperator  Operator=~=
  Relational Operator1 : RelationalOperator  Operator=~=
  Relational Operator2 : RelationalOperator  Operator=>=
  Sum : Sum  Inputs=++  SaturateOnIntegerOverflow=on
  Sum1 : Sum  Inputs=-+  SaturateOnIntegerOverflow=on
  Sum2 : Sum  Inputs=+-  SaturateOnIntegerOverflow=on
  Sum3 : Sum  Inputs=++  SaturateOnIntegerOverflow=on
  Sum4 : Sum  Inputs=++  SaturateOnIntegerOverflow=on
  Switch : Switch  Threshold=eps
  Switch1 : Switch  Threshold=eps
  Switch2 : Switch  Threshold=eps
  Switch: map torque : Switch  Threshold=eps
  T closed throttle : Lookup  InputValues=fc_map_spd*fc_spd_scale  OutputValues=fc_ct_trq*fc_trq_scale
  T_max : Lookup  InputValues=fc_map_spd*fc_spd_scale  OutputValues=fc_max_trq*fc_trq_scale
  alpha : Gain  Gain=1/(fc_inertia+eps)  Multiplication=Element-wise(K.*u)  SaturateOnIntegerOverflow=on
  clutch disengaged : RelationalOperator  Operator===
  dt : Subsystem
      settings: RTWFcnNameOpts=Auto  RTWFileNameOpts=Auto
  effect of inertia (Nm) : Subsystem
      settings: RTWFcnNameOpts=Auto  RTWFileNameOpts=Auto
  just started spin-down/spin-up : Subsystem
      settings: RTWFcnNameOpts=Auto  RTWFileNameOpts=Auto
  no-lag Reset Integrator : Subsystem  mask(No-lag Reset Integrator){@1=vc_idle_spd}
      mask prompts: @1 "Initial Value"
      mask help: No-lag Reset Integrator
      mask init:
      | initval=@1;
      settings: RTWFcnNameOpts=Auto  RTWFileNameOpts=Auto
      mask Help: Integrates first input using Euler technique.\nAt the time step that input 2 <> zero,\noutput is reset to input 3.
      mask Display: disp('1/s\nw/ reset\nno lag')
  Out1 : Outport  Port=1
  tag scope: fc_spd_limited=scoped
  wires:
  IC1/1 -> Logical Operator/1
  Memory4/1 -> Product/1
  [acc_mech_trq_est] -> Sum2/2, Sum4/2
  Product/1 -> Switch/1
  [veh_spd_a_rec_prev] -> Sum/1, Switch/2
  Constant1/1 -> Switch/3
  IC/1 -> Switch1/1
  Constant/1 -> Sum/2
  [cyc_mph_r_prev] -> Sum1/2
  [mpha_prev] -> Gain/1, Sum1/1
  Constant2/1 -> Relational/2
  Sum1/1 -> Relational/1
  Relational/1 -> IC1/1
  Switch/1 -> IC/1
  Gain/1 -> Product/2
  Sum/1 -> Product/3
  Relational Operator/1 -> Logical Operator/2
  Constant3/1 -> Relational Operator/2
  Sum2/1 -> alpha/1
  dt/1(out_1) -> Product1/2
  Product1/1 -> Sum3/1
  alpha/1 -> Product1/1, no-lag Reset Integrator/1(in_1)
  Constant5/1 -> clutch disengaged/2
  Switch1/1 -> Switch2/1
  clutch disengaged/1 -> Logical Operator2/1, just started spin-down/spin-up/1(state)
  [clutch_state] -> Relational Operator/1, clutch disengaged/1
  Memory3/1 -> Sum3/2, Relational Operator2/2, T_max/1, effect of inertia (Nm)/2(prev spd), T closed throttle/1
  <= max spd/1 -> Relational Operator1/2, MinMax1/1
  [engine_on] -> Product2/2
  Constant4/1 -> Product2/1
  MinMax1/1 -> Out1/1, Memory3/1
  Product2/1 -> MinMax1/2
  Switch2/1 -> <= max spd/1, Relational Operator1/1
  Memory2/1 -> Logical Operator1/2
  Logical Operator1/1 -> [fc_spd_limited]
  Relational Operator1/1 -> Logical Operator1/1, Memory2/1
  Switch: map torque/1 -> Sum2/1
  Relational Operator2/1 -> Switch: map torque/2
  T closed throttle/1 -> Switch: map torque/3
  MinMax/1 -> Switch: map torque/1
  T_max/1 -> MinMax/1
  Sum4/1 -> MinMax/2
  effect of inertia (Nm)/1((Nm)) -> Sum4/1
  spd command/1 -> Memory4/1, Switch1/3, Relational Operator2/1, effect of inertia (Nm)/1(req'd spd (rad/s))
  Logical Operator2/1 -> Switch2/2
  Logical Operator/1 -> Switch1/2
  no-lag Reset Integrator/1(out_1) -> Switch2/3
  just started spin-down/spin-up/1(trigger) -> no-lag Reset Integrator/2(in_2)
  Sum3/1 -> no-lag Reset Integrator/3(in_3)

== system lib_fuel_converter3/fuel converter <fc>/IC Engine Model  &  Interface/ic engine model/engine torque ==
  fc_trq_out_r : Inport  Port=1  LatchInput=off
  spd command : Inport  Port=2  LatchInput=off
  engine spd : Inport  Port=3  LatchInput=off
  Block NOTES : Subsystem
      settings: RTWFcnNameOpts=Auto  RTWFileNameOpts=Auto
      mask Display: disp('Block\nNOTES')
  Constant1 : Constant  Value=0
  Constant3 : Constant  Value=1
  Logical Operator : Logic  Operator=OR  Inputs=2
  MinMax : MinMax  Function=min  Inputs=2
  MinMax1 : MinMax  Function=max  Inputs=2
  Sum : Sum  Inputs=++  SaturateOnIntegerOverflow=on
  Sum1 : Sum  Inputs=+-  SaturateOnIntegerOverflow=on
  Switch : Switch  Threshold=eps
  Switch1 : Switch  Threshold=eps
  T_closed throttle : Subsystem
      settings: RTWFcnNameOpts=Auto  RTWFileNameOpts=Auto
  T_max : Subsystem
      settings: RTWFcnNameOpts=Auto  RTWFileNameOpts=Auto
  clutch not disengaged : RelationalOperator  Operator=~=
  effect of inertia (Nm) : Subsystem
      settings: RTWFcnNameOpts=Auto  RTWFileNameOpts=Auto
  engine commanded not to decelerate : RelationalOperator  Operator=<=
  limited : RelationalOperator  Operator=~=
  map torque (Nm) : Outport  Port=1
  torque to shaft (Nm) : Outport  Port=2
  tag scope: fc_trq_limited=scoped
  wires:
  Constant1/1 -> Switch1/3
  Sum1/1 -> Switch1/1
  Switch1/1 -> torque to shaft (Nm)/1
  [clutch_state] -> clutch not disengaged/1
  Constant3/1 -> clutch not disengaged/2
  engine commanded not to decelerate/1 -> Logical Operator/1
  Sum/1 -> Switch/1
  Logical Operator/1 -> Switch/2
  limited/1 -> [fc_trq_limited]
  MinMax/1 -> MinMax1/1
  T_max/1(T_max) -> MinMax/2
  T_closed throttle/1(T_closed throttle) -> Switch/3, MinMax1/2
  MinMax1/1 -> limited/2, map torque (Nm)/1, Sum1/1
  Switch/1 -> MinMax/1, limited/1
  clutch not disengaged/1 -> Switch1/2, Logical Operator/2
  engine spd/1 -> T_closed throttle/1(w_APU), T_max/1(w_APU), engine commanded not to decelerate/1, effect of inertia (Nm)/1(engine spd (rad/s))
  fc_trq_out_r/1 -> Sum/1
  effect of inertia (Nm)/1((Nm)) -> Sum/2, Sum1/2
  spd command/1 -> engine commanded not to decelerate/2

== system lib_fuel_converter3/fuel converter <fc>/IC Engine Model  &  Interface/ic engine model/enhancedToWorkspace ==
  In1 : Inport  Port=1  LatchInput=off
  To Workspace : ToWorkspace  VariableName=fc_spd_out_r  SampleTime=-1  SaveFormat=Array
  wires:
  In1/1 -> To Workspace/1

== system lib_fuel_converter3/fuel converter <fc>/IC Engine Model  &  Interface/ic engine model/enhancedToWorkspace1 ==
  In1 : Inport  Port=1  LatchInput=off
  To Workspace : ToWorkspace  VariableName=fc_spd_est  SampleTime=-1  SaveFormat=Array
  wires:
  In1/1 -> To Workspace/1

== system lib_fuel_converter3/fuel converter <fc>/IC Engine Model  &  Interface/ic engine model/enhancedToWorkspace3 ==
  In1 : Inport  Port=1  LatchInput=off
  To Workspace : ToWorkspace  VariableName=fc_fuel  SampleTime=-1  SaveFormat=Array
  wires:
  In1/1 -> To Workspace/1

== system lib_fuel_converter3/fuel converter <fc>/IC Engine Model  &  Interface/ic engine model/enhancedToWorkspace4 ==
  In1 : Inport  Port=1  LatchInput=off
  To Workspace : ToWorkspace  VariableName=fc_spd_out_a  SampleTime=-1  SaveFormat=Array
  wires:
  In1/1 -> To Workspace/1

== system lib_fuel_converter3/fuel converter <fc>/IC Engine Model  &  Interface/ic engine model/enhancedToWorkspace5 ==
  In1 : Inport  Port=1  LatchInput=off
  To Workspace : ToWorkspace  VariableName=fc_trq_out_a  SampleTime=-1  SaveFormat=Array
  wires:
  In1/1 -> To Workspace/1

== system lib_fuel_converter3/fuel converter <fc>/IC Engine Model  &  Interface/ic engine model/enhancedToWorkspace6 ==
  In1 : Inport  Port=1  LatchInput=off
  To Workspace : ToWorkspace  VariableName=fc_trq_out_r  SampleTime=-1  SaveFormat=Array
  wires:
  In1/1 -> To Workspace/1

== system lib_fuel_converter3/fuel converter <fc>/IC Engine Model  &  Interface/ic engine model/enhancedToWorkspace7 ==
  In1 : Inport  Port=1  LatchInput=off
  To Workspace : ToWorkspace  VariableName=fc_brake_trq  SampleTime=-1  SaveFormat=Array
  wires:
  In1/1 -> To Workspace/1

== system lib_fuel_converter3/fuel converter <fc>/IC Engine Model  &  Interface/ic engine model/fuel use and EO emis Configurable Subsystem ==
  T (Nm) : Inport  Port=1  LatchInput=off
  w (rad/s) : Inport  Port=2  LatchInput=off
  fuel use and EO emis : lib_fuel_converter3/configurable subsystems/fuel use and EO emis
      settings: RTWFcnNameOpts=Auto  RTWFileNameOpts=Auto
  cumulative fuel  use (gal) : Outport  Port=1
  "FC ON?, EOem, MFex, Tex, O2ex" : Outport  Port=2
  Vv,Tfc : Outport  Port=3
  wires:
  fuel use and EO emis/3 -> Vv,Tfc/1
  fuel use and EO emis/2 -> "FC ON?, EOem, MFex, Tex, O2ex"/1
  fuel use and EO emis/1 -> cumulative fuel  use (gal)/1
  w (rad/s)/1 -> fuel use and EO emis/2
  T (Nm)/1 -> fuel use and EO emis/1

== system lib_fuel_converter3/fuel converter <fc>/IC Engine Model  &  Interface/ic engine model/help ==

== system lib_fuel_converter3/fuel converter <fc> no fuel at negative torque/IC Engine Model  &  Interface/ic engine model/Block NOTES ==
  note: This block models the internal combustion engine, and includes inertia effects,
      | performance limits, accessory loads, and temperature transient effects on fuel
      | use, engine-out emissions, and catalyst efficiency.  There are 'leads' to the
      | engine controller here, which controller determines whether the engine is on.

== system lib_fuel_converter3/fuel converter <fc> no fuel at negative torque/IC Engine Model  &  Interface/ic engine model/Speed Limits ==
  Speed Requested : Inport  Port=1  LatchInput=off
  Constant : Constant  Value=0
  Speed Limits : Saturate  UpperLimit=max(fc_map_spd)*fc_spd_scale  LowerLimit=vc_idle_spd*vc_idle_bool  LinearizeAsGain=on
  "if engine is not on, speed is zero" : Switch  Threshold=0.5
  Limited Speed Request : Outport  Port=1
  wires:
  Speed Requested/1 -> Speed Limits/1
  Speed Limits/1 -> "if engine is not on, speed is zero"/1
  "if engine is not on, speed is zero"/1 -> Limited Speed Request/1
  [engine_on] -> "if engine is not on, speed is zero"/2
  Constant/1 -> "if engine is not on, speed is zero"/3
